simulink model "myadc_lib"  (R2013a)
settings: Solver=ode45  StartTime=0.0  StopTime=10e-05  RelTol=1e-3
libraries: mylib x1, dsparch4 x1
settings Model: Creator=bbhattac  LastModifiedBy=bbhattac
settings OptimizationCC: ExpressionDepthLimit=2147483647
settings DebuggingCC: ParameterPrecisionLossMsg=none  FcnCallInpInsideContextMsg=UseLocalSettings
settings GRTTargetCC: CombineOutputUpdateFcns=off  GRTInterface=on

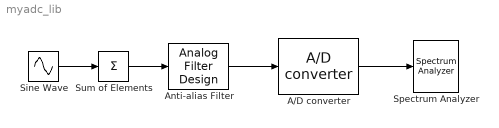
== system myadc_lib ==
  A/D converter : mylib/A//D converter  minDelay=1.0e-09  maxDelay=15.0e-09  nonlingain=0.2  nbits=8
  Anti-alias Filter : dsparch4/Analog Filter Design  method=Butterworth  filttype=Lowpass  N=8  Wlo=2*pi*50e+06  Whi=80  Rp=2  Rs=40
  Sine Wave : Sin  Amplitude=.25  Frequency=2*pi*[20 22]*1e6  SampleTime=0
  Spectrum Analyzer : SpectrumAnalyzer
      settings: CopyFcn=scopeextensions.ScopeBlock.callback(gcbh, 'onBlockCopy', gcbh);  DeleteFcn=scopeextensions.ScopeBlock.callback(gcbh, 'onBlockDelete');  PreSaveFcn=scopeextensions.ScopeBlock.callback(gcbh, 'onModelSave');  NameChangeFcn=scopeextensions.ScopeBlock.callback(gcbh, 'onBlockRename');  CloseFcn=scopeextensions.ScopeBlock.callback(gcbh, 'onBlockClose');  PreDeleteFcn=scopeextensions.ScopeBlock.callback(gcbh, 'onBlockPreDelete');
  Sum of Elements : Sum  Inputs=+
  wires:
  Sine Wave/1 -> Sum of Elements/1
  Sum of Elements/1 -> Anti-alias Filter/1
  Anti-alias Filter/1 -> A/D converter/1
  A/D converter/1 -> Spectrum Analyzer/1
